simulink model "graphml_test_cases"  (R2017b)
settings: Solver=VariableStepAuto  StartTime=0.0  StopTime=10.0  RelTol=1e-3
libraries: simulink x8
settings Model: Creator=cyarp  LastModifiedBy=cyarp

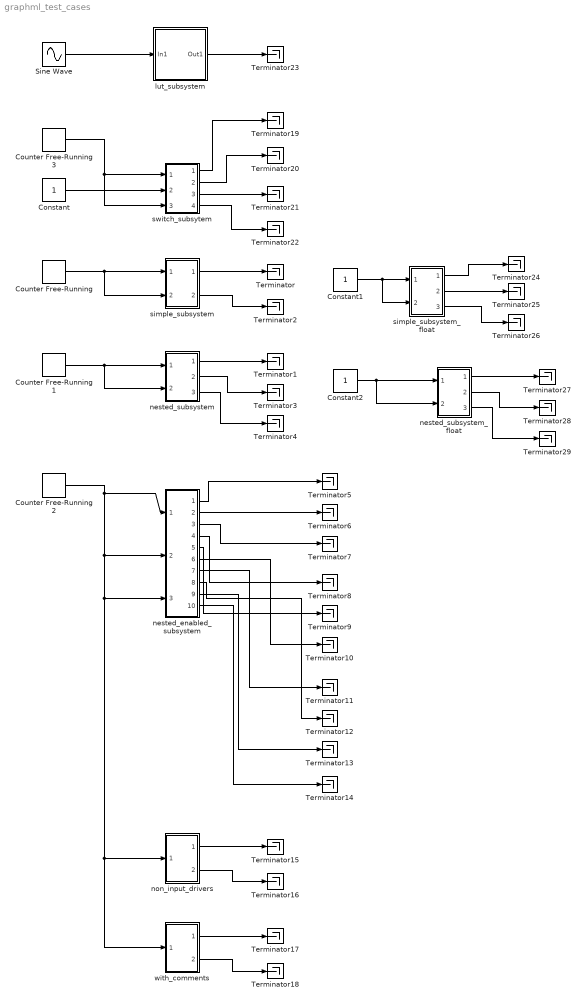
== system graphml_test_cases ==
  Constant : Constant
  Constant1 : Constant
  Constant2 : Constant
  Counter Free-Running{,1..3} (4 alike) : simulink/Sources/Counter Free-Running  NumBits=16  tsamp=-1
  Sine Wave : Sin  Amplitude=4  SampleTime=0
  Terminator{,1..29} (30 alike) : Terminator
  lut_subsystem : Subsystem
  nested_enabled_subsystem : Subsystem
  nested_subsystem : Subsystem
  nested_subsystem_float : Subsystem
  non_input_drivers : Subsystem
  simple_subsystem : Subsystem
  simple_subsystem_float : Subsystem
  switch_subsytem : Subsystem
  with_comments : Subsystem
  wires:
  Counter Free-Running/1 -> simple_subsystem/2(In2), simple_subsystem/1(In1)
  simple_subsystem/1(Out1) -> Terminator/1
  nested_subsystem/1(Out1) -> Terminator1/1
  Counter Free-Running1/1 -> nested_subsystem/2(In2), nested_subsystem/1(In1)
  simple_subsystem/2(Out2) -> Terminator2/1
  nested_subsystem/2(Out2) -> Terminator3/1
  nested_subsystem/3(Out3) -> Terminator4/1
  nested_enabled_subsystem/3(Out2) -> Terminator7/1
  nested_enabled_subsystem/1(Out1) -> Terminator5/1
  nested_enabled_subsystem/2(Out4) -> Terminator6/1
  Counter Free-Running2/1 -> with_comments/1(In1), non_input_drivers/1(In1), nested_enabled_subsystem/3(In3), nested_enabled_subsystem/2(In2), nested_enabled_subsystem/1(In1)
  nested_enabled_subsystem/4(Out3) -> Terminator8/1
  nested_enabled_subsystem/5(Out5) -> Terminator9/1
  nested_enabled_subsystem/6(Out6) -> Terminator10/1
  nested_enabled_subsystem/7(Out7) -> Terminator11/1
  nested_enabled_subsystem/8(Out8) -> Terminator12/1
  nested_enabled_subsystem/9(Out9) -> Terminator13/1
  nested_enabled_subsystem/10(Out10) -> Terminator14/1
  non_input_drivers/1(Out1) -> Terminator15/1
  non_input_drivers/2(Out2) -> Terminator16/1
  with_comments/1(Out1) -> Terminator17/1
  with_comments/2(Out2) -> Terminator18/1
  switch_subsytem/2(Out2) -> Terminator20/1
  Counter Free-Running3/1 -> switch_subsytem/3(In3), switch_subsytem/1(In1)
  switch_subsytem/1(Out1) -> Terminator19/1
  switch_subsytem/3(Out3) -> Terminator21/1
  switch_subsytem/4(Out4) -> Terminator22/1
  Sine Wave/1 -> lut_subsystem/1(In1)
  lut_subsystem/1(Out1) -> Terminator23/1
  Constant/1 -> switch_subsytem/2(In2)
  simple_subsystem_float/2(Out2) -> Terminator25/1
  simple_subsystem_float/1(Out1) -> Terminator24/1
  Constant1/1 -> simple_subsystem_float/2(In2), simple_subsystem_float/1(In1)
  simple_subsystem_float/3(Out3) -> Terminator26/1
  nested_subsystem_float/2(Out2) -> Terminator28/1
  Constant2/1 -> nested_subsystem_float/2(In2), nested_subsystem_float/1(In1)
  nested_subsystem_float/1(Out1) -> Terminator27/1
  nested_subsystem_float/3(Out3) -> Terminator29/1

== system graphml_test_cases/lut_subsystem ==
  In1 : Inport
  1-D Lookup Table : Lookup_n-D  NumberOfTableDimensions=1  BreakpointsForDimension1=[-5:5]  IndexSearchMethod=Evenly spaced points  Table=atan([-5:5])  InterpMethod=Flat  InternalRulePriority=Speed  RndMeth=Simplest  InputSameDT=on
  Out1 : Outport
  wires:
  1-D Lookup Table/1 -> Out1/1
  In1/1 -> 1-D Lookup Table/1

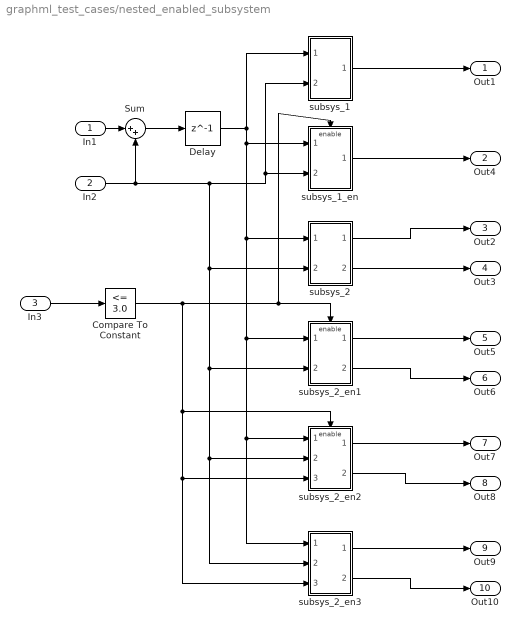
== system graphml_test_cases/nested_enabled_subsystem ==
  In1 : Inport
  In2 : Inport  Port=2
  In3 : Inport  Port=3
  Compare To Constant : simulink/Logic and Bit Operations/Compare To Constant  relop=<=  const=3.0  OutDataTypeStr=boolean
  Delay : Delay  DelayLength=1  InitialCondition=0
  Sum : Sum  Inputs=|++
  subsys_1 : Subsystem
  subsys_1_en : Subsystem
  subsys_2 : Subsystem
  subsys_2_en1 : Subsystem
  subsys_2_en2 : Subsystem
  subsys_2_en3 : Subsystem
  Out1 : Outport
  Out4 : Outport  Port=2
  Out2 : Outport  Port=3
  Out3 : Outport  Port=4
  Out5 : Outport  Port=5
  Out6 : Outport  Port=6
  Out7 : Outport  Port=7
  Out8 : Outport  Port=8
  Out9 : Outport  Port=9
  Out10 : Outport  Port=10
  wires:
  In1/1 -> Sum/1
  Sum/1 -> Delay/1
  Delay/1 -> subsys_1_en/1(In1), subsys_2_en3/1(In1), subsys_2_en2/1(In1), subsys_2_en1/1(In1), subsys_2/1(In1), subsys_1/1(In1)
  subsys_1/1(Out1) -> Out1/1
  In2/1 -> subsys_2_en3/2(In2), subsys_2_en2/2(In2), subsys_2_en1/2(In2), subsys_2/2(In2), subsys_1_en/2(In2), subsys_1/2(In2), Sum/2
  subsys_2/1(Out1) -> Out2/1
  subsys_2/2(Out2) -> Out3/1
  subsys_1_en/1(Out1) -> Out4/1
  In3/1 -> Compare To Constant/1
  Compare To Constant/1 -> subsys_2_en3/3(In3), subsys_2_en2/3(In3), subsys_2_en2/Enable, subsys_1_en/Enable, subsys_2_en1/Enable
  subsys_2_en1/1(Out1) -> Out5/1
  subsys_2_en1/2(Out2) -> Out6/1
  subsys_2_en2/1(Out1) -> Out7/1
  subsys_2_en2/2(Out2) -> Out8/1
  subsys_2_en3/1(Out1) -> Out9/1
  subsys_2_en3/2(Out2) -> Out10/1

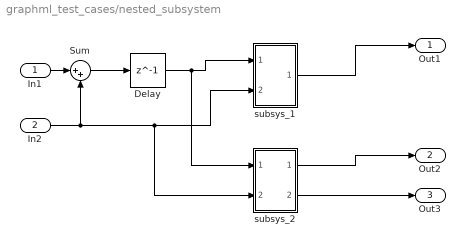
== system graphml_test_cases/nested_subsystem ==
  In1 : Inport
  In2 : Inport  Port=2
  Delay : Delay  DelayLength=1  InitialCondition=0
  Sum : Sum  Inputs=|++
  subsys_1 : Subsystem
  subsys_2 : Subsystem
  Out1 : Outport
  Out2 : Outport  Port=2
  Out3 : Outport  Port=3
  wires:
  In1/1 -> Sum/1
  Sum/1 -> Delay/1
  Delay/1 -> subsys_2/1(In1), subsys_1/1(In1)
  subsys_1/1(Out1) -> Out1/1
  In2/1 -> subsys_2/2(In2), subsys_1/2(In2), Sum/2
  subsys_2/1(Out1) -> Out2/1
  subsys_2/2(Out2) -> Out3/1

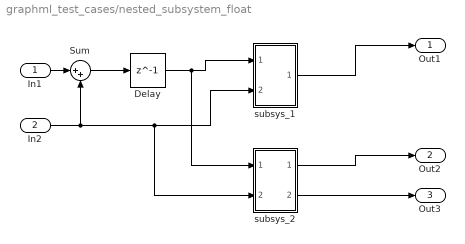
== system graphml_test_cases/nested_subsystem_float ==
  In1 : Inport
  In2 : Inport  Port=2
  Delay : Delay  DelayLength=1  InitialCondition=0
  Sum : Sum  Inputs=|++
  subsys_1 : Subsystem
  subsys_2 : Subsystem
  Out1 : Outport
  Out2 : Outport  Port=2
  Out3 : Outport  Port=3
  wires:
  In1/1 -> Sum/1
  Sum/1 -> Delay/1
  Delay/1 -> subsys_2/1(In1), subsys_1/1(In1)
  subsys_1/1(Out1) -> Out1/1
  In2/1 -> subsys_2/2(In2), subsys_1/2(In2), Sum/2
  subsys_2/1(Out1) -> Out2/1
  subsys_2/2(Out2) -> Out3/1

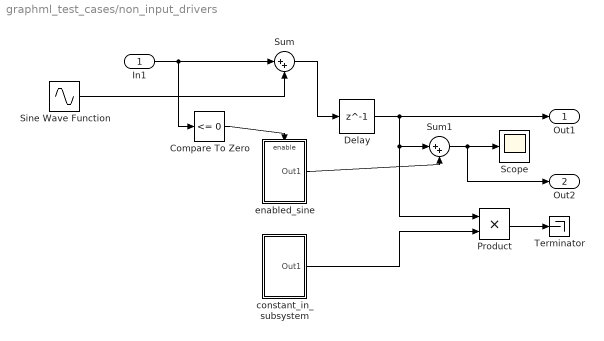
== system graphml_test_cases/non_input_drivers ==
  In1 : Inport
  Compare To Zero : simulink/Logic and Bit Operations/Compare To Zero  relop=<=  OutDataTypeStr=boolean
  Delay : Delay  DelayLength=1  InitialCondition=0
  Product : Product
  Scope : Scope
  Sine Wave Function : Sin  SampleTime=0
  Sum : Sum  Inputs=|++
  Sum1 : Sum  Inputs=|++
  Terminator : Terminator
  constant_in_subsystem : Subsystem
  enabled_sine : Subsystem
  Out1 : Outport
  Out2 : Outport  Port=2
  wires:
  In1/1 -> Compare To Zero/1, Sum/1
  Sum/1 -> Delay/1
  Delay/1 -> Product/1, Sum1/1, Out1/1
  Sum1/1 -> Out2/1, Scope/1
  Product/1 -> Terminator/1
  Sine Wave Function/1 -> Sum/2
  constant_in_subsystem/1(Out1) -> Product/2
  enabled_sine/1(Out1) -> Sum1/2
  Compare To Zero/1 -> enabled_sine/Enable

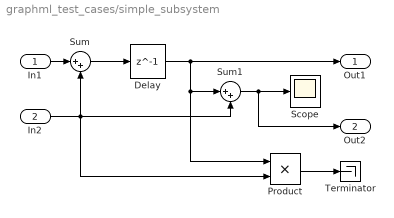
== system graphml_test_cases/simple_subsystem ==
  In1 : Inport
  In2 : Inport  Port=2
  Delay : Delay  DelayLength=1  InitialCondition=0
  Product : Product
  Scope : Scope
  Sum : Sum  Inputs=|++
  Sum1 : Sum  Inputs=|++
  Terminator : Terminator
  Out1 : Outport
  Out2 : Outport  Port=2
  wires:
  In1/1 -> Sum/1
  Sum/1 -> Delay/1
  Delay/1 -> Product/1, Sum1/1, Out1/1
  In2/1 -> Product/2, Sum1/2, Sum/2
  Sum1/1 -> Out2/1, Scope/1
  Product/1 -> Terminator/1

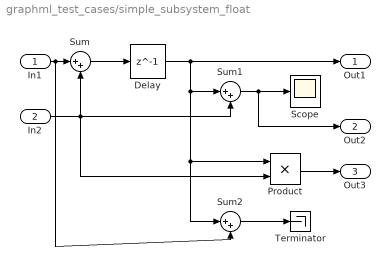
== system graphml_test_cases/simple_subsystem_float ==
  In1 : Inport
  In2 : Inport  Port=2
  Delay : Delay  DelayLength=1  InitialCondition=0
  Product : Product
  Scope : Scope
  Sum : Sum  Inputs=|++
  Sum1 : Sum  Inputs=|++
  Sum2 : Sum  Inputs=|++
  Terminator : Terminator
  Out1 : Outport
  Out2 : Outport  Port=2
  Out3 : Outport  Port=3
  wires:
  In1/1 -> Sum2/2, Sum/1
  Sum/1 -> Delay/1
  Delay/1 -> Sum2/1, Product/1, Sum1/1, Out1/1
  In2/1 -> Product/2, Sum1/2, Sum/2
  Sum1/1 -> Out2/1, Scope/1
  Product/1 -> Out3/1
  Sum2/1 -> Terminator/1

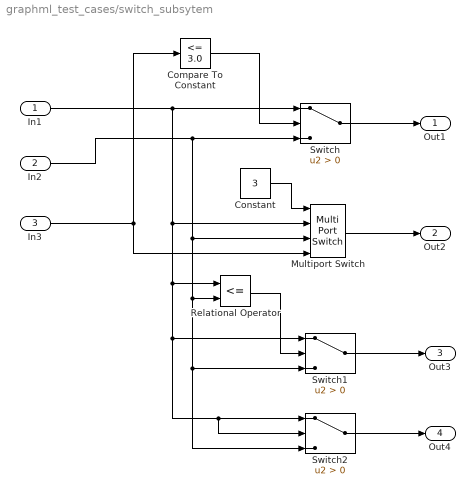
== system graphml_test_cases/switch_subsytem ==
  In1 : Inport
  In2 : Inport  Port=2
  In3 : Inport  Port=3
  Compare To Constant : simulink/Logic and Bit Operations/Compare To Constant  relop=<=  const=3.0  OutDataTypeStr=boolean
  Constant : Constant  Value=3
  Multiport Switch : MultiPortSwitch
  Relational Operator : RelationalOperator  Operator=<=  OutDataTypeStr=boolean  RndMeth=Simplest
  Switch : Switch  Criteria=u2 > Threshold
  Switch1 : Switch  Criteria=u2 > Threshold
  Switch2 : Switch  Criteria=u2 > Threshold
  Out1 : Outport
  Out2 : Outport  Port=2
  Out3 : Outport  Port=3
  Out4 : Outport  Port=4
  wires:
  In1/1 -> Relational Operator/1, Switch2/2, Switch2/1, Switch1/1, Multiport Switch/2, Switch/1
  In3/1 -> Multiport Switch/4, Compare To Constant/1
  In2/1 -> Switch/3, Multiport Switch/3, Relational Operator/2, Switch2/3, Switch1/3
  Constant/1 -> Multiport Switch/1
  Switch/1 -> Out1/1
  Compare To Constant/1 -> Switch/2
  Multiport Switch/1 -> Out2/1
  Switch1/1 -> Out3/1
  Relational Operator/1 -> Switch1/2
  Switch2/1 -> Out4/1

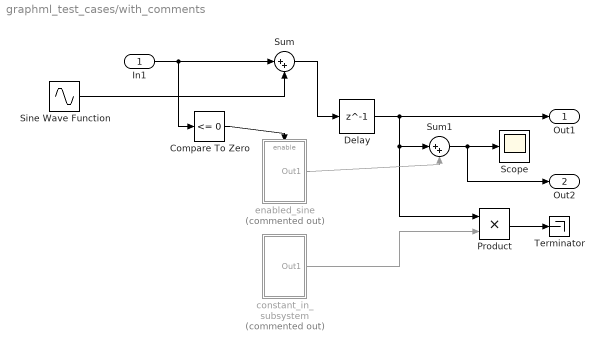
== system graphml_test_cases/with_comments ==
  In1 : Inport
  Compare To Zero : simulink/Logic and Bit Operations/Compare To Zero  relop=<=  OutDataTypeStr=boolean
  Delay : Delay  DelayLength=1  InitialCondition=0
  Product : Product
  Scope : Scope
  Sine Wave Function : Sin  SampleTime=0
  Sum : Sum  Inputs=|++
  Sum1 : Sum  Inputs=|++
  Terminator : Terminator
  constant_in_subsystem : Subsystem  Commented=on
  enabled_sine : Subsystem  Commented=on
  Out1 : Outport
  Out2 : Outport  Port=2
  wires:
  In1/1 -> Compare To Zero/1, Sum/1
  Sum/1 -> Delay/1
  Delay/1 -> Product/1, Sum1/1, Out1/1
  Sum1/1 -> Out2/1, Scope/1
  Product/1 -> Terminator/1
  Sine Wave Function/1 -> Sum/2
  constant_in_subsystem/1(Out1) -> Product/2
  enabled_sine/1(Out1) -> Sum1/2
  Compare To Zero/1 -> enabled_sine/Enable

== system graphml_test_cases/nested_enabled_subsystem/subsys_1 ==
  In1 : Inport
  In2 : Inport  Port=2
  Delay1 : Delay  DelayLength=1  InitialCondition=0
  Product : Product
  Out1 : Outport
  wires:
  Delay1/1 -> Out1/1
  In2/1 -> Product/2
  In1/1 -> Product/1
  Product/1 -> Delay1/1

== system graphml_test_cases/nested_enabled_subsystem/subsys_1_en ==
  In1 : Inport
  In2 : Inport  Port=2
  Enable : EnablePort
  Delay1 : Delay  DelayLength=1  InitialCondition=0
  Product : Product
  Out1 : Outport
  wires:
  Delay1/1 -> Out1/1
  In2/1 -> Product/2
  In1/1 -> Product/1
  Product/1 -> Delay1/1

== system graphml_test_cases/nested_enabled_subsystem/subsys_2 ==
  In1 : Inport
  In2 : Inport  Port=2
  Delay1 : Delay  DelayLength=1  InitialCondition=0
  Product : Product
  sub_sub_sys : Subsystem
  Out1 : Outport
  Out2 : Outport  Port=2
  wires:
  Delay1/1 -> sub_sub_sys/1(In1), Out1/1
  In2/1 -> sub_sub_sys/2(In2), Product/2
  In1/1 -> Product/1
  Product/1 -> Delay1/1
  sub_sub_sys/1(Out1) -> Out2/1

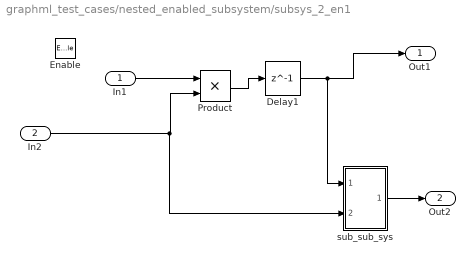
== system graphml_test_cases/nested_enabled_subsystem/subsys_2_en1 ==
  In1 : Inport
  In2 : Inport  Port=2
  Enable : EnablePort
  Delay1 : Delay  DelayLength=1  InitialCondition=0
  Product : Product
  sub_sub_sys : Subsystem
  Out1 : Outport
  Out2 : Outport  Port=2
  wires:
  Delay1/1 -> sub_sub_sys/1(In1), Out1/1
  In2/1 -> sub_sub_sys/2(In2), Product/2
  In1/1 -> Product/1
  Product/1 -> Delay1/1
  sub_sub_sys/1(Out1) -> Out2/1

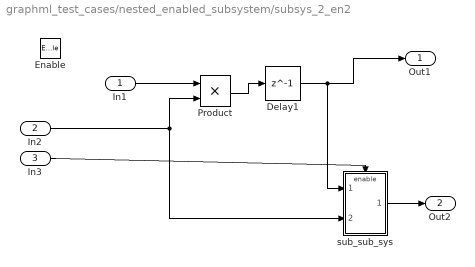
== system graphml_test_cases/nested_enabled_subsystem/subsys_2_en2 ==
  In1 : Inport
  In2 : Inport  Port=2
  In3 : Inport  Port=3
  Enable : EnablePort
  Delay1 : Delay  DelayLength=1  InitialCondition=0
  Product : Product
  sub_sub_sys : Subsystem
  Out1 : Outport
  Out2 : Outport  Port=2
  wires:
  Delay1/1 -> sub_sub_sys/1(In1), Out1/1
  In2/1 -> sub_sub_sys/2(In2), Product/2
  In1/1 -> Product/1
  Product/1 -> Delay1/1
  sub_sub_sys/1(Out1) -> Out2/1
  In3/1 -> sub_sub_sys/Enable

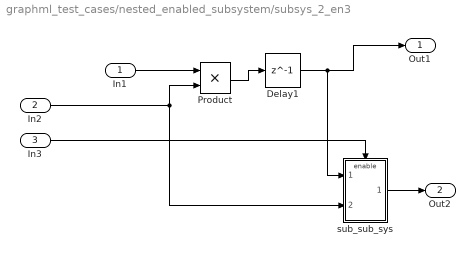
== system graphml_test_cases/nested_enabled_subsystem/subsys_2_en3 ==
  In1 : Inport
  In2 : Inport  Port=2
  In3 : Inport  Port=3
  Delay1 : Delay  DelayLength=1  InitialCondition=0
  Product : Product
  sub_sub_sys : Subsystem
  Out1 : Outport
  Out2 : Outport  Port=2
  wires:
  Delay1/1 -> sub_sub_sys/1(In1), Out1/1
  In2/1 -> sub_sub_sys/2(In2), Product/2
  In1/1 -> Product/1
  Product/1 -> Delay1/1
  sub_sub_sys/1(Out1) -> Out2/1
  In3/1 -> sub_sub_sys/Enable

== system graphml_test_cases/nested_subsystem/subsys_1 ==
  In1 : Inport
  In2 : Inport  Port=2
  Delay1 : Delay  DelayLength=1  InitialCondition=0
  Product : Product
  Out1 : Outport
  wires:
  Delay1/1 -> Out1/1
  In2/1 -> Product/2
  In1/1 -> Product/1
  Product/1 -> Delay1/1

== system graphml_test_cases/nested_subsystem/subsys_2 ==
  In1 : Inport
  In2 : Inport  Port=2
  Delay1 : Delay  DelayLength=1  InitialCondition=0
  Product : Product
  sub_sub_sys : Subsystem
  Out1 : Outport
  Out2 : Outport  Port=2
  wires:
  Delay1/1 -> sub_sub_sys/1(In1), Out1/1
  In2/1 -> sub_sub_sys/2(In2), Product/2
  In1/1 -> Product/1
  Product/1 -> Delay1/1
  sub_sub_sys/1(Out1) -> Out2/1

== system graphml_test_cases/nested_subsystem_float/subsys_1 ==
  In1 : Inport
  In2 : Inport  Port=2
  Delay1 : Delay  DelayLength=1  InitialCondition=0
  Product : Product
  Out1 : Outport
  wires:
  Delay1/1 -> Out1/1
  In2/1 -> Product/2
  In1/1 -> Product/1
  Product/1 -> Delay1/1

== system graphml_test_cases/nested_subsystem_float/subsys_2 ==
  In1 : Inport
  In2 : Inport  Port=2
  Delay1 : Delay  DelayLength=1  InitialCondition=0
  Product : Product
  sub_sub_sys : Subsystem
  Out1 : Outport
  Out2 : Outport  Port=2
  wires:
  Delay1/1 -> sub_sub_sys/1(In1), Out1/1
  In2/1 -> sub_sub_sys/2(In2), Product/2
  In1/1 -> Product/1
  Product/1 -> Delay1/1
  sub_sub_sys/1(Out1) -> Out2/1

== system graphml_test_cases/non_input_drivers/constant_in_subsystem ==
  Constant : Constant
  Out1 : Outport
  wires:
  Constant/1 -> Out1/1

== system graphml_test_cases/non_input_drivers/enabled_sine ==
  Enable : EnablePort
  Sine Wave Function : Sin  SampleTime=0
  Out1 : Outport
  wires:
  Sine Wave Function/1 -> Out1/1

== system graphml_test_cases/with_comments/constant_in_subsystem ==
  Constant : Constant
  Out1 : Outport
  wires:
  Constant/1 -> Out1/1

== system graphml_test_cases/with_comments/enabled_sine ==
  Enable : EnablePort
  Sine Wave Function : Sin  SampleTime=0
  Out1 : Outport
  wires:
  Sine Wave Function/1 -> Out1/1

== system graphml_test_cases/nested_enabled_subsystem/subsys_2/sub_sub_sys ==
  In1 : Inport
  In2 : Inport  Port=2
  Delay1 : Delay  DelayLength=1  InitialCondition=0
  Product : Product
  Out1 : Outport
  wires:
  Delay1/1 -> Out1/1
  In2/1 -> Product/2
  In1/1 -> Product/1
  Product/1 -> Delay1/1

== system graphml_test_cases/nested_enabled_subsystem/subsys_2_en1/sub_sub_sys ==
  In1 : Inport
  In2 : Inport  Port=2
  Delay1 : Delay  DelayLength=1  InitialCondition=0
  Product : Product
  Out1 : Outport
  wires:
  Delay1/1 -> Out1/1
  In2/1 -> Product/2
  In1/1 -> Product/1
  Product/1 -> Delay1/1

== system graphml_test_cases/nested_enabled_subsystem/subsys_2_en2/sub_sub_sys ==
  In1 : Inport
  In2 : Inport  Port=2
  Enable : EnablePort
  Delay1 : Delay  DelayLength=1  InitialCondition=0
  Product : Product
  Out1 : Outport
  wires:
  Delay1/1 -> Out1/1
  In2/1 -> Product/2
  In1/1 -> Product/1
  Product/1 -> Delay1/1

== system graphml_test_cases/nested_enabled_subsystem/subsys_2_en3/sub_sub_sys ==
  In1 : Inport
  In2 : Inport  Port=2
  Enable : EnablePort
  Delay1 : Delay  DelayLength=1  InitialCondition=0
  Product : Product
  Out1 : Outport
  wires:
  Delay1/1 -> Out1/1
  In2/1 -> Product/2
  In1/1 -> Product/1
  Product/1 -> Delay1/1

== system graphml_test_cases/nested_subsystem/subsys_2/sub_sub_sys ==
  In1 : Inport
  In2 : Inport  Port=2
  Delay1 : Delay  DelayLength=1  InitialCondition=0
  Product : Product
  Out1 : Outport
  wires:
  Delay1/1 -> Out1/1
  In2/1 -> Product/2
  In1/1 -> Product/1
  Product/1 -> Delay1/1

== system graphml_test_cases/nested_subsystem_float/subsys_2/sub_sub_sys ==
  In1 : Inport
  In2 : Inport  Port=2
  Delay1 : Delay  DelayLength=1  InitialCondition=0
  Product : Product
  Out1 : Outport
  wires:
  Delay1/1 -> Out1/1
  In2/1 -> Product/2
  In1/1 -> Product/1
  Product/1 -> Delay1/1
